simulink model "assumed_mode_ppo_simulink"  (R2025b)
settings: Solver=ode4  StartTime=0.0  StopTime=10  FixedStep=0.002  RelTol=1e-3
values from neighbouring files (symbols this model uses):
  par = [ ... (first row only)    [build_ppo_parameter_vector.m]    (also in run_assumed_mode.m; test_ppo_ps2f_simulink.m = build_ppo_parameter_vector(p,Ts,2); test_ppo_simulink.m = build_ppo_parameter_vector(p,Ts,2); train_ppo_simulink.m = build_ppo_parameter_vector(p,Ts,2))
  tau_prev0 = 0    [test_ppo_ps2f_simulink.m]    (also in test_ppo_simulink.m; train_ppo_simulink.m; trained_mep_ppo.mat)
  Ts = par(32)    [ppo_evaluate_agent.m]    (also in ppo_reward.m; run_assumed_mode.m = 0.02; test_ppo_ps2f_simulink.m = p.sim.Ts; test_ppo_simulink.m = S.Ts)
  x_prev0 = x0    [test_ppo_ps2f_simulink.m]    (also in test_ppo_simulink.m; train_ppo_simulink.m; trained_mep_ppo.mat = [0 0 0 0 0 0])
libraries: rllib x1
settings Model: Creator=Nargiz  LastModifiedBy=Nargiz

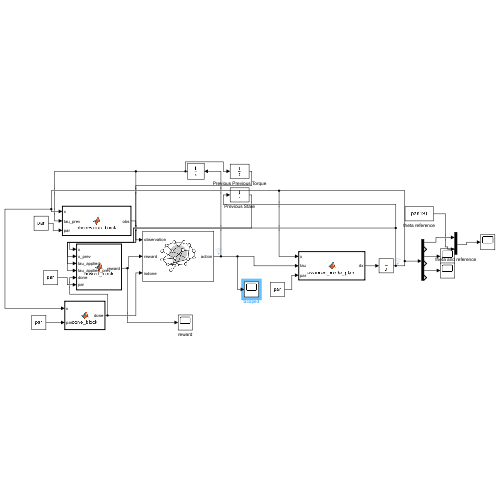
[thumbnail: Simulink's stored preview of the top-level diagram]
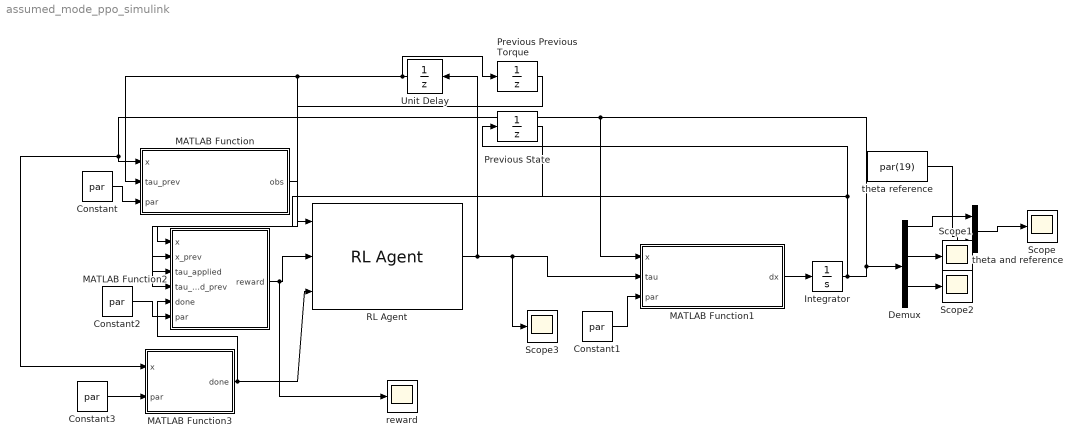
== system assumed_mode_ppo_simulink ==
  Constant{,1..3} (4 alike) : Constant  Value=par
  Demux : Demux  Outputs=6
  Integrator : Integrator
  MATLAB Function : MATLAB Function  TreatAsAtomicUnit=on  SystemSampleTime=Ts
  MATLAB Function1 : MATLAB Function  TreatAsAtomicUnit=on
  MATLAB Function2 : MATLAB Function  TreatAsAtomicUnit=on  SystemSampleTime=Ts
  MATLAB Function3 : MATLAB Function  TreatAsAtomicUnit=on  SystemSampleTime=Ts
  Previous Previous Torque : UnitDelay  InitialCondition=tau_prev0  SampleTime=Ts  HasFrameUpgradeWarning=on
  Previous State : UnitDelay  InitialCondition=x_prev0  SampleTime=Ts  HasFrameUpgradeWarning=on
  RL Agent : rllib/RL Agent  Agent=agentObj  ExternalActionAsInput=off  ProvideLastAction=off  ProvideCumRwd=off  TreatAsDirectFeedthrough=on  UseStrictObservationDataTypes=off
  Scope{,1..3} (4 alike) : Scope
      Scope settings: ActiveDisplayYMinimum=-0.069710536173875834  ActiveDisplayYMaximum=0.62739482556488269
      Scope1 settings: ActiveDisplayYMinimum=-0.009692971347242875  ActiveDisplayYMaximum=0.0061296856285213384  DataLoggingVariableName=ScopeData2
      Scope2 settings: ActiveDisplayYMinimum=-0.00094209526231751688  ActiveDisplayYMaximum=0.0012706451074967976  DataLoggingVariableName=ScopeData3
      Scope3 settings: ActiveDisplayYMinimum=-0.10213103611022234  ActiveDisplayYMaximum=0.37039362359791994  DataLoggingVariableName=ScopeData4
  Unit Delay : UnitDelay  InitialCondition=tau_prev0  SampleTime=Ts  HasFrameUpgradeWarning=on
  reward : Scope
  theta and reference : Mux  Inputs=2
  theta reference : Constant  Value=par(19)
  wires:
  MATLAB Function1/1(dx) -> Integrator/1
  Integrator/1 -> Previous State/1, MATLAB Function2/1(x), MATLAB Function1/1(x), MATLAB Function/1(x), MATLAB Function3/1(x), Demux/1
  Constant1/1 -> MATLAB Function1/3(par)
  Constant/1 -> MATLAB Function/3(par)
  MATLAB Function2/1(reward) -> reward/1, RL Agent/2
  Constant3/1 -> MATLAB Function3/2(par)
  Demux/3 -> Scope1/1
  Demux/5 -> Scope2/1
  Unit Delay/1 -> MATLAB Function/2(tau_prev), MATLAB Function2/3(tau_applied), Previous Previous Torque/1
  Previous State/1 -> MATLAB Function2/2(x_prev)
  Previous Previous Torque/1 -> MATLAB Function2/4(tau_applied_prev)
  MATLAB Function3/1(done) -> MATLAB Function2/5(done), RL Agent/3
  Constant2/1 -> MATLAB Function2/6(par)
  MATLAB Function/1(obs) -> RL Agent/1
  RL Agent/1 -> Scope3/1, MATLAB Function1/2(tau), Unit Delay/1
  Demux/1 -> theta and reference/1
  theta reference/1 -> theta and reference/2
  theta and reference/1 -> Scope/1

== matlab function assumed_mode_ppo_simulink/MATLAB Function1 ==
  data: x input; tau input; dx output; par input
function dx = assumed_mode_plant(x, tau, par)

%#codegen

dx = zeros(6,1);  

%% Unpack parameter vector
l       = par(2);
J2      = par(3);
mr      = par(4);
mp      = par(5);
Btheta  = par(6);

phi1L   = par(7);
phi2L   = par(8);
phi1pL  = par(9);
phi2pL  = par(10);

Meta1   = par(11);
Meta2   = par(12);
Keta1   = par(13);
Keta2   = par(14);
Deta1   = par(15);
Deta2   = par(16);

tau_max = par(21);

%% States
theta     = x(1);
theta_dot = x(2);

eta1      = x(3);
eta1_dot  = x(4);

eta2      = x(5);
eta2_dot  = x(6);

qdot = [theta_dot; eta1_dot; eta2_dot];

%% Torque saturation
tau = max(min(tau, tau_max), -tau_max);

%% Tip deflection and tip slope
alpha = phi1pL*eta1 + phi2pL*eta2;
gamma = theta + alpha;

gvec = [1; phi1pL; phi2pL];
wvec = [0; phi1L; phi2L];

%% Rigid link and payload coefficients
Ir = mr*l^2/3;
Ip = mp*l^2;

Arot = Ir + Ip;
Mvert = mr + mp;
Across = mr*l/2 + mp*l;

%% Mass matrix
M = zeros(3,3);

M(1,1) = M(1,1) + J2;
M(2,2) = M(2,2) + Meta1;
M(3,3) = M(3,3) + Meta2;

M = M ...
    + Arot*(gvec*gvec') ...
    + Mvert*(wvec*wvec') ...
    + Across*cos(gamma)*(gvec*wvec' + wvec*gvec');

%% Nonlinear velocity terms
dM = zeros(3,3,3);

common_dM_dgamma = -Across*sin(gamma)*(gvec*wvec' + wvec*gvec');

for kk = 1:3
    dM(:,:,kk) = common_dM_dgamma * gvec(kk);
end

h = zeros(3,1);

for ii = 1:3
    for jj = 1:3
        for kk = 1:3
            Gamma_ijk = 0.5*(dM(ii,jj,kk) + dM(ii,kk,jj) - dM(jj,kk,ii));
            h(ii) = h(ii) + Gamma_ijk*qdot(jj)*qdot(kk);
        end
    end
end

%% Stiffness and damping
Kq = [0;
      Keta1*eta1;
      Keta2*eta2];

Dq = [Btheta*theta_dot;
      Deta1*eta1_dot;
      Deta2*eta2_dot];

Q = [tau; 0; 0];

%% Solve dynamics
qdd = M \ (Q - h - Dq - Kq);

%% Output derivative
dx(1) = theta_dot;
dx(2) = qdd(1);

dx(3) = eta1_dot;
dx(4) = qdd(2);

dx(5) = eta2_dot;
dx(6) = qdd(3);

end

== matlab function assumed_mode_ppo_simulink/MATLAB Function ==
  data: x input; tau_prev input; obs output; par input
function obs = observation_block(x,tau_prev,par)
%#codegen
obs = zeros(12,1);
obs = ppo_observation(x,tau_prev,par);
end

== matlab function assumed_mode_ppo_simulink/MATLAB Function2 ==
  data: x input; reward output; x_prev input; tau_applied input; tau_applied_prev input; done input; par input
function reward = reward_block(x,x_prev,tau_applied,tau_applied_prev,done,par)
%#codegen
reward = 0.0;
reward = ppo_reward(x,x_prev,tau_applied,tau_applied_prev,done,par);
end

== matlab function assumed_mode_ppo_simulink/MATLAB Function3 ==
  data: x input; done output; par input
function done = done_block(x,par)
%#codegen
done = false;
done = ppo_done(x,par);
end
